simulink model "simulink_discrete_controller_model"  (R2019b)
settings: Solver=VariableStepAuto  StartTime=0.0  StopTime=200e-3  MaxStep=100e-6  RelTol=1e-3
undefined symbols (not defined in the file or in its folder): ki, kp
libraries: cstblocks x3, simulink x1
settings Model: Creator=dvarx  LastModifiedBy=dvarx
settings SFSimCC: CustomCodeUndefinedFunction=UseInterfaceOnly

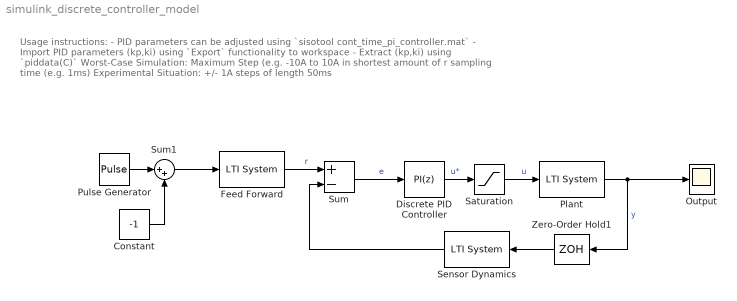
== system simulink_discrete_controller_model ==
  note: Usage instructions:
      |
      | - PID parameters can be adjusted using `sisotool cont_time_pi_controller.mat`
      | - Import PID parameters (kp,ki) using `Export` functionality to workspace
      | - Extract (kp,ki) using `piddata(C)`
      |
      | Worst-Case Simulation: Maximum Step (e.g. -10A to 10A in shortest amount of r sampling time (e.g. 1ms)
      | Experimental Situation: +/- 1A steps of length 50ms
  Constant : Constant  Value=-1
  Discrete PID Controller : simulink/Continuous/PID Controller  Controller=PI  Form=Parallel  TimeDomain=Discrete-time  SampleTime=-1  IntegratorMethod=Forward Euler  FilterMethod=Forward Euler  ControllerParametersSource=internal  P=kp  I=ki  D=0  UseFilter=on  N=100  TunerSelectOption=Transfer Function Based (PID Tuner App)  InitialConditionSource=internal  InitialConditionForIntegrator=0  InitialConditionForFilter=0  DifferentiatorICPrevScaledInput=0  ExternalReset=none  TrackingMode=off  Kt=1  LimitOutput=off  UpperSaturationLimit=inf  LowerSaturationLimit=-inf  LinearizeAsGain=off  AntiWindupMode=none  Kb=1  POutMin=[]  POutMax=[]  IOutMin=[]  IOutMax=[]  DOutMin=[]  DOutMax=[]  NOutMin=[]  NOutMax=[]  SumOutMin=[]  SumOutMax=[]  SaturationOutMin=[]  SaturationOutMax=[]  PParamMin=[]  PParamMax=[]  IParamMin=[]  IParamMax=[]  DParamMin=[]  DParamMax=[]  NParamMin=[]  NParamMax=[]  KbParamMin=[]  KbParamMax=[]  KtParamMin=[]  KtParamMax=[]  KbOutMin=[]  KbOutMax=[]  KtOutMin=[]  KtOutMax=[]  IntegratorOutMin=[]  IntegratorOutMax=[]  FilterOutMin=[]  FilterOutMax=[]  SumI1OutMin=[]  SumI1OutMax=[]  SumI2OutMin=[]  SumI2OutMax=[]  SumI3OutMin=[]  SumI3OutMax=[]  SumI4OutMin=[]  SumI4OutMax=[]  SumDOutMin=[]  SumDOutMax=[]  DifferentiatorOutMin=[]  DifferentiatorOutMax=[]  FilterDiffOutCoefMin=[]  FilterDiffOutCoefMax=[]  ReciprocalOutMin=[]  ReciprocalOutMax=[]  SumDenOutMin=[]  SumDenOutMax=[]  SumNumOutMin=[]  SumNumOutMax=[]  DivideOutMin=[]  DivideOutMax=[]  IntegratorContinuousStateAttributes=''  IntegratorStateMustResolveToSignalObject=off  IntegratorRTWStateStorageClass=Auto  FilterContinuousStateAttributes=''  FilterStateMustResolveToSignalObject=off  FilterRTWStateStorageClass=Auto  ParallelPVariant=InternalParameters  IdealPVariant=Disabled  IVariant=InternalParameters  DVariant=Disabled  IntegratorVariant=Discrete  SatVariant=Disabled  AWVariant=Passthrough  PCopyVariant=Disabled  TRVariant=Disabled  FdbkBlocksVariant=Forward  IdealPFdbkVariant=Disabled  SatFdbkVariant=Disabled  DerivativeFilterVariant=Disabled  NVariant=Disabled  NCopyVariant=Disabled_SignalSpec  FilterICVariant=Disabled  IntegratorICVariant=InternalICs  ExternalResetVariant=Disabled  TRSumVariant=Passthrough  SumFdbkVariant=Disabled  SumVariant=Sum_PI
  Feed Forward : cstblocks/LTI System  sys=F  IC=[]
  Output : Scope
  Plant : cstblocks/LTI System  sys=G  IC=[]
  Pulse Generator : DiscretePulseGenerator  PulseType=Time based  Amplitude=2  Period=50e-3  PulseWidth=50
  Saturation : Saturate  UpperLimit=30  LowerLimit=-30
  Sensor Dynamics : cstblocks/LTI System  sys=H  IC=[]
  Sum : Sum  Inputs=+-  SaturateOnIntegerOverflow=on  InputSameDT=on  OutDataTypeStr=Inherit: Same as first input
  Sum1 : Sum  Inputs=|++
  Zero-Order Hold1 : ZeroOrderHold  SampleTime=200e-6
  wires:
  Feed Forward/1 -> Sum/1  "r"
  Sensor Dynamics/1 -> Sum/2
  Sum/1 -> Discrete PID Controller/1  "e"
  Plant/1 -> Zero-Order Hold1/1, Output/1  "y"
  Zero-Order Hold1/1 -> Sensor Dynamics/1
  Discrete PID Controller/1 -> Saturation/1  "u*"
  Saturation/1 -> Plant/1  "u"
  Sum1/1 -> Feed Forward/1
  Pulse Generator/1 -> Sum1/1
  Constant/1 -> Sum1/2
